simulink model "Telescope_model_PID"  (R2024b)
settings: Solver=ode4  StartTime=0.0  StopTime=SimulationTime  FixedStep=Tc  RelTol=1e-5
undefined symbols (not defined in the file): Arcs2Deg, Deg2Arcs, Kd_az, Kd_el, Ki_az, Ki_el, Kp_az, Kp_el, Kv, Prepocessor, Scenario, sgn, sysAz, sysEL, VonKarman
libraries: simulink x16
(part 2 of 2)

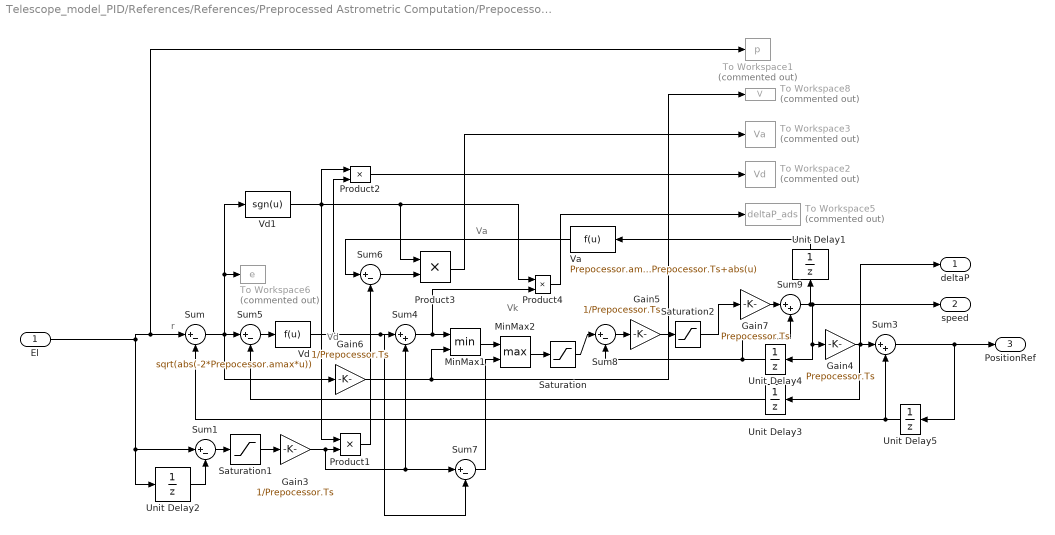
== system Telescope_model_PID/References/References/Preprocessed Astrometric Computation/Prepocessor Elavation/Prepocessor Elevation ==
  note: Vd
  note: Va
  note: Vk
  note: r
  El : Inport
  Gain3 : Gain  Gain=1/Prepocessor.Ts
  Gain4 : Gain  Gain=Prepocessor.Ts
  Gain5 : Gain  Gain=1/Prepocessor.Ts
  Gain6 : Gain  Gain=1/Prepocessor.Ts
  Gain7 : Gain  Gain=Prepocessor.Ts
  MinMax1 : MinMax  Inputs=2
  MinMax2 : MinMax  Function=max  Inputs=2
  Product{1..4} (4 alike) : Product
  Saturation : Saturate  UpperLimit=Prepocessor.vmax  LowerLimit=-Prepocessor.vmax
  Saturation1 : Saturate  UpperLimit=Prepocessor.vmax*Prepocessor.Ts  LowerLimit=-Prepocessor.vmax*Prepocessor.Ts
  Saturation2 : Saturate  UpperLimit=Prepocessor.amax  LowerLimit=-Prepocessor.amax
  Sum{,1,5..8} (6 alike) : Sum  Inputs=|+-
  Sum3 : Sum  Inputs=|++
  Sum4 : Sum  Inputs=|++
  Sum9 : Sum  Inputs=|++
  To Workspace1 : ToWorkspace  Commented=on  VariableName=p  SampleTime=-1
  To Workspace2 : ToWorkspace  Commented=on  VariableName=Vd  SampleTime=-1
  To Workspace3 : ToWorkspace  Commented=on  VariableName=Va  SampleTime=-1
  To Workspace5 : ToWorkspace  Commented=on  VariableName=deltaP_ads  SampleTime=-1
  To Workspace6 : ToWorkspace  Commented=on  VariableName=e  SampleTime=-1
  To Workspace8 : ToWorkspace  Commented=on  VariableName=V  SampleTime=-1
  Unit Delay{1..4} (4 alike) : UnitDelay  SampleTime=-1  HasFrameUpgradeWarning=on
  Unit Delay5 : UnitDelay  InitialCondition=Prepocessor.p0el  SampleTime=-1  HasFrameUpgradeWarning=on
  Va : Fcn  Expr=Prepocessor.amax*Prepocessor.Ts+abs(u)
  Vd : Fcn  Expr=sqrt(abs(-2*Prepocessor.amax*u))
  Vd1 : Fcn  Expr=sgn(u)
  deltaP : Outport
  speed : Outport  Port=2
  PositionRef : Outport  Port=3
  wires:
  Unit Delay5/1 -> Sum/2, Sum3/2
  Product4/1 -> To Workspace5/1
  El/1 -> Unit Delay2/1, Sum1/1, Sum/1, To Workspace1/1
  Product2/1 -> To Workspace2/1
  Product3/1 -> To Workspace3/1
  Vd/1 -> Product2/2, Sum7/2, Sum4/1
  Sum4/1 -> Product4/2, MinMax1/1
  Unit Delay3/1 -> Sum5/2
  Product1/1 -> Sum6/2
  Gain4/1 -> deltaP/1, Sum3/1, Unit Delay3/1
  Vd1/1 -> Product2/1, Product1/1, Product4/1, Product3/1
  Saturation2/1 -> Gain7/1
  Sum7/1 -> MinMax2/2
  Va/1 -> Sum6/1
  Sum1/1 -> Saturation1/1
  Sum/1 -> Sum5/1, Gain6/1, Vd1/1, To Workspace6/1
  Unit Delay2/1 -> Sum1/2
  Gain7/1 -> Sum9/1
  Sum9/1 -> speed/1, Unit Delay4/1, Gain4/1, Unit Delay1/1
  Unit Delay4/1 -> Sum8/2, Sum9/2
  Gain6/1 -> MinMax1/2, To Workspace8/1
  MinMax1/1 -> MinMax2/1
  Gain3/1 -> Sum7/1, Sum4/2, Product1/2
  Sum6/1 -> Product3/2
  Saturation1/1 -> Gain3/1
  Saturation/1 -> Sum8/1
  Sum8/1 -> Gain5/1
  Sum5/1 -> Vd/1
  MinMax2/1 -> Saturation/1
  Unit Delay1/1 -> Va/1
  Gain5/1 -> Saturation2/1
  Sum3/1 -> Unit Delay5/1, PositionRef/1

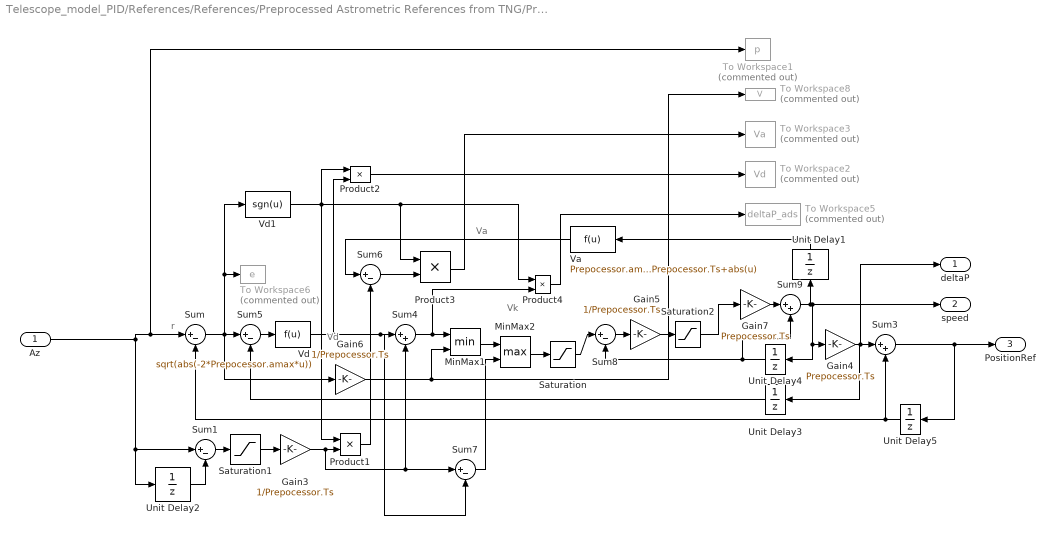
== system Telescope_model_PID/References/References/Preprocessed Astrometric References from TNG/Prepocessor Azimuth/Prepocessor Elevation ==
  note: Vd
  note: Va
  note: Vk
  note: r
  Az : Inport
  Gain3 : Gain  Gain=1/Prepocessor.Ts
  Gain4 : Gain  Gain=Prepocessor.Ts
  Gain5 : Gain  Gain=1/Prepocessor.Ts
  Gain6 : Gain  Gain=1/Prepocessor.Ts
  Gain7 : Gain  Gain=Prepocessor.Ts
  MinMax1 : MinMax  Inputs=2
  MinMax2 : MinMax  Function=max  Inputs=2
  Product{1..4} (4 alike) : Product
  Saturation : Saturate  UpperLimit=Prepocessor.vmax  LowerLimit=-Prepocessor.vmax
  Saturation1 : Saturate  UpperLimit=Prepocessor.vmax*Prepocessor.Ts  LowerLimit=-Prepocessor.vmax*Prepocessor.Ts
  Saturation2 : Saturate  UpperLimit=Prepocessor.amax  LowerLimit=-Prepocessor.amax
  Sum{,1,5..8} (6 alike) : Sum  Inputs=|+-
  Sum3 : Sum  Inputs=|++
  Sum4 : Sum  Inputs=|++
  Sum9 : Sum  Inputs=|++
  To Workspace1 : ToWorkspace  Commented=on  VariableName=p  SampleTime=-1
  To Workspace2 : ToWorkspace  Commented=on  VariableName=Vd  SampleTime=-1
  To Workspace3 : ToWorkspace  Commented=on  VariableName=Va  SampleTime=-1
  To Workspace5 : ToWorkspace  Commented=on  VariableName=deltaP_ads  SampleTime=-1
  To Workspace6 : ToWorkspace  Commented=on  VariableName=e  SampleTime=-1
  To Workspace8 : ToWorkspace  Commented=on  VariableName=V  SampleTime=-1
  Unit Delay{1..4} (4 alike) : UnitDelay  SampleTime=-1  HasFrameUpgradeWarning=on
  Unit Delay5 : UnitDelay  InitialCondition=Prepocessor.p0az  SampleTime=-1  HasFrameUpgradeWarning=on
  Va : Fcn  Expr=Prepocessor.amax*Prepocessor.Ts+abs(u)
  Vd : Fcn  Expr=sqrt(abs(-2*Prepocessor.amax*u))
  Vd1 : Fcn  Expr=sgn(u)
  deltaP : Outport
  speed : Outport  Port=2
  PositionRef : Outport  Port=3
  wires:
  Unit Delay5/1 -> Sum/2, Sum3/2
  Product4/1 -> To Workspace5/1
  Az/1 -> Unit Delay2/1, Sum1/1, Sum/1, To Workspace1/1
  Product2/1 -> To Workspace2/1
  Product3/1 -> To Workspace3/1
  Vd/1 -> Product2/2, Sum7/2, Sum4/1
  Sum4/1 -> Product4/2, MinMax1/1
  Unit Delay3/1 -> Sum5/2
  Product1/1 -> Sum6/2
  Gain4/1 -> deltaP/1, Sum3/1, Unit Delay3/1
  Vd1/1 -> Product2/1, Product1/1, Product4/1, Product3/1
  Saturation2/1 -> Gain7/1
  Sum7/1 -> MinMax2/2
  Va/1 -> Sum6/1
  Sum1/1 -> Saturation1/1
  Sum/1 -> Sum5/1, Gain6/1, Vd1/1, To Workspace6/1
  Unit Delay2/1 -> Sum1/2
  Gain7/1 -> Sum9/1
  Sum9/1 -> speed/1, Unit Delay4/1, Gain4/1, Unit Delay1/1
  Unit Delay4/1 -> Sum8/2, Sum9/2
  Gain6/1 -> MinMax1/2, To Workspace8/1
  MinMax1/1 -> MinMax2/1
  Gain3/1 -> Sum7/1, Sum4/2, Product1/2
  Sum6/1 -> Product3/2
  Saturation1/1 -> Gain3/1
  Saturation/1 -> Sum8/1
  Sum8/1 -> Gain5/1
  Sum5/1 -> Vd/1
  MinMax2/1 -> Saturation/1
  Unit Delay1/1 -> Va/1
  Gain5/1 -> Saturation2/1
  Sum3/1 -> Unit Delay5/1, PositionRef/1

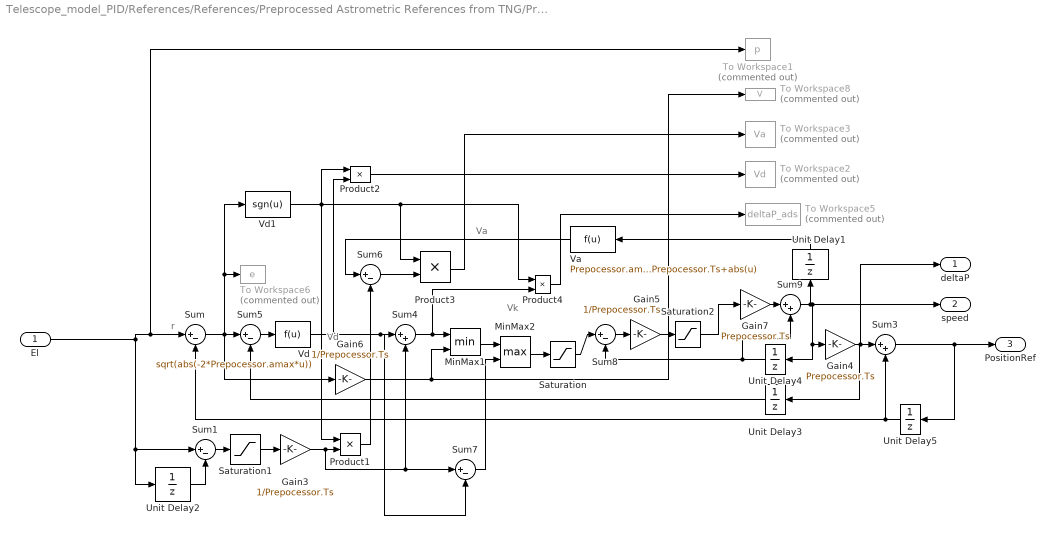
== system Telescope_model_PID/References/References/Preprocessed Astrometric References from TNG/Prepocessor Elavation/Prepocessor Elevation ==
  note: Vd
  note: Va
  note: Vk
  note: r
  El : Inport
  Gain3 : Gain  Gain=1/Prepocessor.Ts
  Gain4 : Gain  Gain=Prepocessor.Ts
  Gain5 : Gain  Gain=1/Prepocessor.Ts
  Gain6 : Gain  Gain=1/Prepocessor.Ts
  Gain7 : Gain  Gain=Prepocessor.Ts
  MinMax1 : MinMax  Inputs=2
  MinMax2 : MinMax  Function=max  Inputs=2
  Product{1..4} (4 alike) : Product
  Saturation : Saturate  UpperLimit=Prepocessor.vmax  LowerLimit=-Prepocessor.vmax
  Saturation1 : Saturate  UpperLimit=Prepocessor.vmax*Prepocessor.Ts  LowerLimit=-Prepocessor.vmax*Prepocessor.Ts
  Saturation2 : Saturate  UpperLimit=Prepocessor.amax  LowerLimit=-Prepocessor.amax
  Sum{,1,5..8} (6 alike) : Sum  Inputs=|+-
  Sum3 : Sum  Inputs=|++
  Sum4 : Sum  Inputs=|++
  Sum9 : Sum  Inputs=|++
  To Workspace1 : ToWorkspace  Commented=on  VariableName=p  SampleTime=-1
  To Workspace2 : ToWorkspace  Commented=on  VariableName=Vd  SampleTime=-1
  To Workspace3 : ToWorkspace  Commented=on  VariableName=Va  SampleTime=-1
  To Workspace5 : ToWorkspace  Commented=on  VariableName=deltaP_ads  SampleTime=-1
  To Workspace6 : ToWorkspace  Commented=on  VariableName=e  SampleTime=-1
  To Workspace8 : ToWorkspace  Commented=on  VariableName=V  SampleTime=-1
  Unit Delay{1..4} (4 alike) : UnitDelay  SampleTime=-1  HasFrameUpgradeWarning=on
  Unit Delay5 : UnitDelay  InitialCondition=Prepocessor.p0el  SampleTime=-1  HasFrameUpgradeWarning=on
  Va : Fcn  Expr=Prepocessor.amax*Prepocessor.Ts+abs(u)
  Vd : Fcn  Expr=sqrt(abs(-2*Prepocessor.amax*u))
  Vd1 : Fcn  Expr=sgn(u)
  deltaP : Outport
  speed : Outport  Port=2
  PositionRef : Outport  Port=3
  wires:
  Unit Delay5/1 -> Sum/2, Sum3/2
  Product4/1 -> To Workspace5/1
  El/1 -> Unit Delay2/1, Sum1/1, Sum/1, To Workspace1/1
  Product2/1 -> To Workspace2/1
  Product3/1 -> To Workspace3/1
  Vd/1 -> Product2/2, Sum7/2, Sum4/1
  Sum4/1 -> Product4/2, MinMax1/1
  Unit Delay3/1 -> Sum5/2
  Product1/1 -> Sum6/2
  Gain4/1 -> deltaP/1, Sum3/1, Unit Delay3/1
  Vd1/1 -> Product2/1, Product1/1, Product4/1, Product3/1
  Saturation2/1 -> Gain7/1
  Sum7/1 -> MinMax2/2
  Va/1 -> Sum6/1
  Sum1/1 -> Saturation1/1
  Sum/1 -> Sum5/1, Gain6/1, Vd1/1, To Workspace6/1
  Unit Delay2/1 -> Sum1/2
  Gain7/1 -> Sum9/1
  Sum9/1 -> speed/1, Unit Delay4/1, Gain4/1, Unit Delay1/1
  Unit Delay4/1 -> Sum8/2, Sum9/2
  Gain6/1 -> MinMax1/2, To Workspace8/1
  MinMax1/1 -> MinMax2/1
  Gain3/1 -> Sum7/1, Sum4/2, Product1/2
  Sum6/1 -> Product3/2
  Saturation1/1 -> Gain3/1
  Saturation/1 -> Sum8/1
  Sum8/1 -> Gain5/1
  Sum5/1 -> Vd/1
  MinMax2/1 -> Saturation/1
  Unit Delay1/1 -> Va/1
  Gain5/1 -> Saturation2/1
  Sum3/1 -> Unit Delay5/1, PositionRef/1

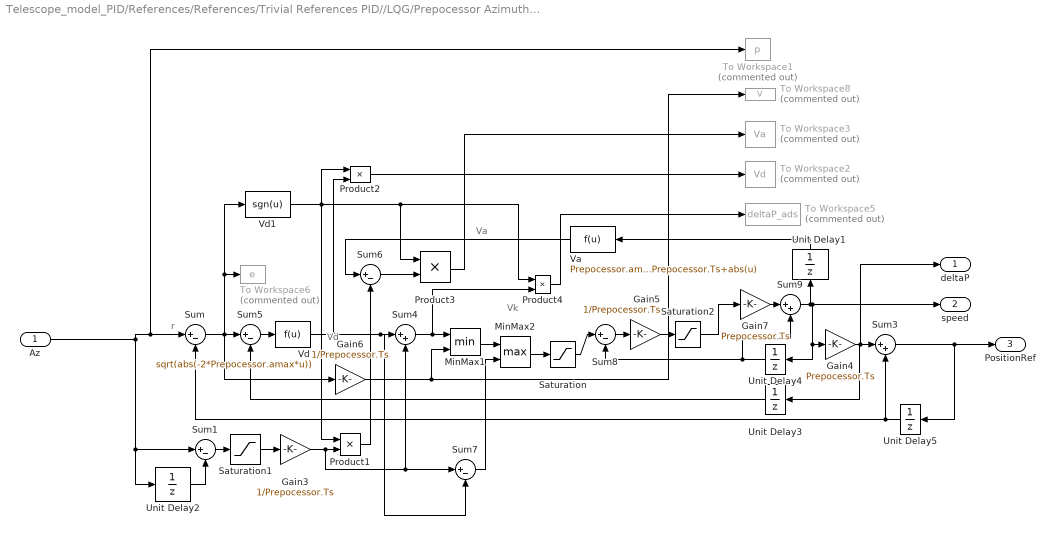
== system Telescope_model_PID/References/References/Trivial References PID//LQG/Prepocessor Azimuth/Prepocessor Elevation ==
  note: Vd
  note: Va
  note: Vk
  note: r
  Az : Inport
  Gain3 : Gain  Gain=1/Prepocessor.Ts
  Gain4 : Gain  Gain=Prepocessor.Ts
  Gain5 : Gain  Gain=1/Prepocessor.Ts
  Gain6 : Gain  Gain=1/Prepocessor.Ts
  Gain7 : Gain  Gain=Prepocessor.Ts
  MinMax1 : MinMax  Inputs=2
  MinMax2 : MinMax  Function=max  Inputs=2
  Product{1..4} (4 alike) : Product
  Saturation : Saturate  UpperLimit=Prepocessor.vmax  LowerLimit=-Prepocessor.vmax
  Saturation1 : Saturate  UpperLimit=Prepocessor.vmax*Prepocessor.Ts  LowerLimit=-Prepocessor.vmax*Prepocessor.Ts
  Saturation2 : Saturate  UpperLimit=Prepocessor.amax  LowerLimit=-Prepocessor.amax
  Sum{,1,5..8} (6 alike) : Sum  Inputs=|+-
  Sum3 : Sum  Inputs=|++
  Sum4 : Sum  Inputs=|++
  Sum9 : Sum  Inputs=|++
  To Workspace1 : ToWorkspace  Commented=on  VariableName=p  SampleTime=-1
  To Workspace2 : ToWorkspace  Commented=on  VariableName=Vd  SampleTime=-1
  To Workspace3 : ToWorkspace  Commented=on  VariableName=Va  SampleTime=-1
  To Workspace5 : ToWorkspace  Commented=on  VariableName=deltaP_ads  SampleTime=-1
  To Workspace6 : ToWorkspace  Commented=on  VariableName=e  SampleTime=-1
  To Workspace8 : ToWorkspace  Commented=on  VariableName=V  SampleTime=-1
  Unit Delay{1..4} (4 alike) : UnitDelay  SampleTime=-1  HasFrameUpgradeWarning=on
  Unit Delay5 : UnitDelay  InitialCondition=Prepocessor.p0az  SampleTime=-1  HasFrameUpgradeWarning=on
  Va : Fcn  Expr=Prepocessor.amax*Prepocessor.Ts+abs(u)
  Vd : Fcn  Expr=sqrt(abs(-2*Prepocessor.amax*u))
  Vd1 : Fcn  Expr=sgn(u)
  deltaP : Outport
  speed : Outport  Port=2
  PositionRef : Outport  Port=3
  wires:
  Unit Delay5/1 -> Sum/2, Sum3/2
  Product4/1 -> To Workspace5/1
  Az/1 -> Unit Delay2/1, Sum1/1, Sum/1, To Workspace1/1
  Product2/1 -> To Workspace2/1
  Product3/1 -> To Workspace3/1
  Vd/1 -> Product2/2, Sum7/2, Sum4/1
  Sum4/1 -> Product4/2, MinMax1/1
  Unit Delay3/1 -> Sum5/2
  Product1/1 -> Sum6/2
  Gain4/1 -> deltaP/1, Sum3/1, Unit Delay3/1
  Vd1/1 -> Product2/1, Product1/1, Product4/1, Product3/1
  Saturation2/1 -> Gain7/1
  Sum7/1 -> MinMax2/2
  Va/1 -> Sum6/1
  Sum1/1 -> Saturation1/1
  Sum/1 -> Sum5/1, Gain6/1, Vd1/1, To Workspace6/1
  Unit Delay2/1 -> Sum1/2
  Gain7/1 -> Sum9/1
  Sum9/1 -> speed/1, Unit Delay4/1, Gain4/1, Unit Delay1/1
  Unit Delay4/1 -> Sum8/2, Sum9/2
  Gain6/1 -> MinMax1/2, To Workspace8/1
  MinMax1/1 -> MinMax2/1
  Gain3/1 -> Sum7/1, Sum4/2, Product1/2
  Sum6/1 -> Product3/2
  Saturation1/1 -> Gain3/1
  Saturation/1 -> Sum8/1
  Sum8/1 -> Gain5/1
  Sum5/1 -> Vd/1
  MinMax2/1 -> Saturation/1
  Unit Delay1/1 -> Va/1
  Gain5/1 -> Saturation2/1
  Sum3/1 -> Unit Delay5/1, PositionRef/1

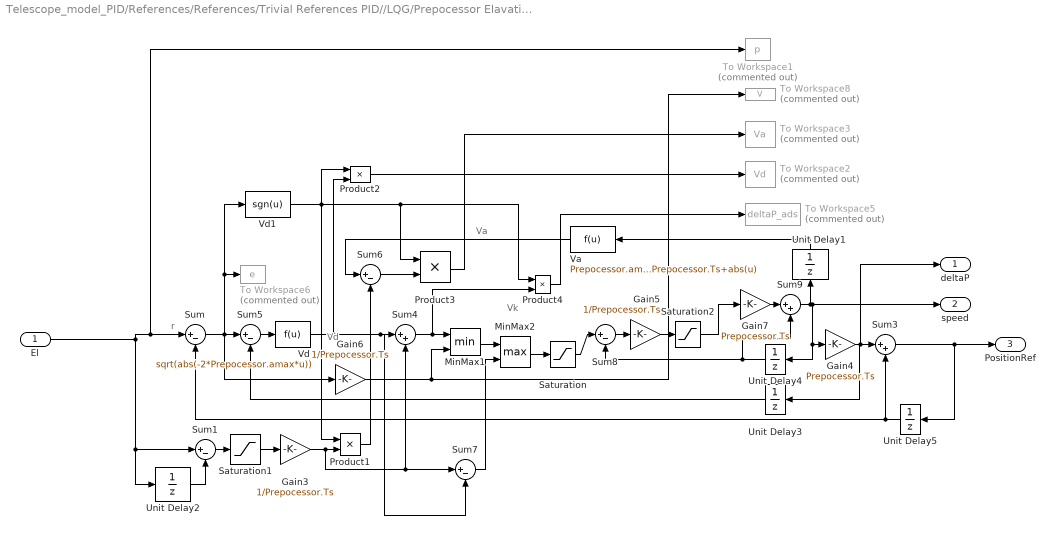
== system Telescope_model_PID/References/References/Trivial References PID//LQG/Prepocessor Elavation/Prepocessor Elevation ==
  note: Vd
  note: Va
  note: Vk
  note: r
  El : Inport
  Gain3 : Gain  Gain=1/Prepocessor.Ts
  Gain4 : Gain  Gain=Prepocessor.Ts
  Gain5 : Gain  Gain=1/Prepocessor.Ts
  Gain6 : Gain  Gain=1/Prepocessor.Ts
  Gain7 : Gain  Gain=Prepocessor.Ts
  MinMax1 : MinMax  Inputs=2
  MinMax2 : MinMax  Function=max  Inputs=2
  Product{1..4} (4 alike) : Product
  Saturation : Saturate  UpperLimit=Prepocessor.vmax  LowerLimit=-Prepocessor.vmax
  Saturation1 : Saturate  UpperLimit=Prepocessor.vmax*Prepocessor.Ts  LowerLimit=-Prepocessor.vmax*Prepocessor.Ts
  Saturation2 : Saturate  UpperLimit=Prepocessor.amax  LowerLimit=-Prepocessor.amax
  Sum{,1,5..8} (6 alike) : Sum  Inputs=|+-
  Sum3 : Sum  Inputs=|++
  Sum4 : Sum  Inputs=|++
  Sum9 : Sum  Inputs=|++
  To Workspace1 : ToWorkspace  Commented=on  VariableName=p  SampleTime=-1
  To Workspace2 : ToWorkspace  Commented=on  VariableName=Vd  SampleTime=-1
  To Workspace3 : ToWorkspace  Commented=on  VariableName=Va  SampleTime=-1
  To Workspace5 : ToWorkspace  Commented=on  VariableName=deltaP_ads  SampleTime=-1
  To Workspace6 : ToWorkspace  Commented=on  VariableName=e  SampleTime=-1
  To Workspace8 : ToWorkspace  Commented=on  VariableName=V  SampleTime=-1
  Unit Delay{1..4} (4 alike) : UnitDelay  SampleTime=-1  HasFrameUpgradeWarning=on
  Unit Delay5 : UnitDelay  InitialCondition=Prepocessor.p0el  SampleTime=-1  HasFrameUpgradeWarning=on
  Va : Fcn  Expr=Prepocessor.amax*Prepocessor.Ts+abs(u)
  Vd : Fcn  Expr=sqrt(abs(-2*Prepocessor.amax*u))
  Vd1 : Fcn  Expr=sgn(u)
  deltaP : Outport
  speed : Outport  Port=2
  PositionRef : Outport  Port=3
  wires:
  Unit Delay5/1 -> Sum/2, Sum3/2
  Product4/1 -> To Workspace5/1
  El/1 -> Unit Delay2/1, Sum1/1, Sum/1, To Workspace1/1
  Product2/1 -> To Workspace2/1
  Product3/1 -> To Workspace3/1
  Vd/1 -> Product2/2, Sum7/2, Sum4/1
  Sum4/1 -> Product4/2, MinMax1/1
  Unit Delay3/1 -> Sum5/2
  Product1/1 -> Sum6/2
  Gain4/1 -> deltaP/1, Sum3/1, Unit Delay3/1
  Vd1/1 -> Product2/1, Product1/1, Product4/1, Product3/1
  Saturation2/1 -> Gain7/1
  Sum7/1 -> MinMax2/2
  Va/1 -> Sum6/1
  Sum1/1 -> Saturation1/1
  Sum/1 -> Sum5/1, Gain6/1, Vd1/1, To Workspace6/1
  Unit Delay2/1 -> Sum1/2
  Gain7/1 -> Sum9/1
  Sum9/1 -> speed/1, Unit Delay4/1, Gain4/1, Unit Delay1/1
  Unit Delay4/1 -> Sum8/2, Sum9/2
  Gain6/1 -> MinMax1/2, To Workspace8/1
  MinMax1/1 -> MinMax2/1
  Gain3/1 -> Sum7/1, Sum4/2, Product1/2
  Sum6/1 -> Product3/2
  Saturation1/1 -> Gain3/1
  Saturation/1 -> Sum8/1
  Sum8/1 -> Gain5/1
  Sum5/1 -> Vd/1
  MinMax2/1 -> Saturation/1
  Unit Delay1/1 -> Va/1
  Gain5/1 -> Saturation2/1
  Sum3/1 -> Unit Delay5/1, PositionRef/1

== system Telescope_model_PID/Telescope Model/Azimuth Model 50 deg/Noise Model/Von Karman Torque PSD/Sv ==
  note: Output PSD
  note: Denominator
  f : Inport
  Add : Sum
  Constant : Constant
  Constant1 : Constant  Value=5/6
  Constant2 : Constant  Value=4*(VonKarman.I*VonKarman.v_mean)^2*(VonKarman.L/VonKarman.v_mean)
  Divide : Product  Inputs=*/
  Gain : Gain  Gain=(1.339*VonKarman.L)/VonKarman.v_mean
  Square : Math  Operator=square
  Square1 : Math  Operator=pow
  Out_Sv : Outport
  wires:
  Constant/1 -> Add/1
  f/1 -> Gain/1
  Gain/1 -> Square/1
  Square/1 -> Add/2
  Add/1 -> Square1/1
  Constant1/1 -> Square1/2
  [DEN] -> Divide/2
  Square1/1 -> [DEN]
  Constant2/1 -> Divide/1
  Divide/1 -> Out_Sv/1

== system Telescope_model_PID/Telescope Model/Azimuth Model 50 deg/Noise Model/Von Karman Torque PSD/X ==
  note: X PSD
  f : Inport
  Add : Sum
  Constant : Constant
  Constant1 : Constant  Value=4/3
  Constant2 : Constant
  Divide : Product  Inputs=*/
  Gain : Gain  Gain=2*sqrt(VonKarman.A)/VonKarman.v_mean
  Square1 : Math  Operator=pow
  Out_X : Outport
  wires:
  Constant/1 -> Add/1
  f/1 -> Gain/1
  Constant1/1 -> Square1/2
  Constant2/1 -> Divide/1
  Divide/1 -> Out_X/1
  Add/1 -> Divide/2
  Gain/1 -> Square1/1
  Square1/1 -> Add/2

== system Telescope_model_PID/Telescope Model/Elevation Model/Noise Model/Von Karman Torque PSD/Sv ==
  note: Output PSD
  note: Denominator
  f : Inport
  Add : Sum
  Constant : Constant
  Constant1 : Constant  Value=5/6
  Constant2 : Constant  Value=4*(VonKarman.I*VonKarman.v_mean)^2*(VonKarman.L/VonKarman.v_mean)
  Divide : Product  Inputs=*/
  Gain : Gain  Gain=(1.339*VonKarman.L)/VonKarman.v_mean
  Square : Math  Operator=square
  Square1 : Math  Operator=pow
  Out_Sv : Outport
  wires:
  Constant/1 -> Add/1
  f/1 -> Gain/1
  Gain/1 -> Square/1
  Square/1 -> Add/2
  Add/1 -> Square1/1
  Constant1/1 -> Square1/2
  [DEN] -> Divide/2
  Square1/1 -> [DEN]
  Constant2/1 -> Divide/1
  Divide/1 -> Out_Sv/1

== system Telescope_model_PID/Telescope Model/Elevation Model/Noise Model/Von Karman Torque PSD/X ==
  note: X PSD
  f : Inport
  Add : Sum
  Constant : Constant
  Constant1 : Constant  Value=4/3
  Constant2 : Constant
  Divide : Product  Inputs=*/
  Gain : Gain  Gain=2*sqrt(VonKarman.A)/VonKarman.v_mean
  Square1 : Math  Operator=pow
  Out_X : Outport
  wires:
  Constant/1 -> Add/1
  f/1 -> Gain/1
  Constant1/1 -> Square1/2
  Constant2/1 -> Divide/1
  Divide/1 -> Out_X/1
  Add/1 -> Divide/2
  Gain/1 -> Square1/1
  Square1/1 -> Add/2

== matlab function Telescope_model_PID/References/References/Astrometric Computation/MATLAB Function ==
  data: clo input; Time input; RAhh input; RAmm input; RAss input; DECdd input; DECmm input; DECss input; Latitude input; Longitude input; VLT input; Az output; Alt output
function [Az, Alt] = astroCalc(clo, Time, RAhh, RAmm, RAss, DECdd, DECmm, DECss, Latitude, Longitude, VLT)

  
   %% Legge l'orario del clock di sistema
   Y = Time(1);
   M = Time(2);
   D = Time(3);
   H = Time(4);
   MN = Time(5);
   S = Time(6);
   S = S + clo;
   if S > 60
       S = 0;
       MN = MN+1;
   end
   if MN>60
       MN = 00;
       H = H+1;
   end
   if H>24
       H = 1;
       D = D+1;
   end
   if D>31
       D = 0;
       M = M+1;
   end
   if M>12
       M = 1;
       Y = Y+1;
   end

   % Calcola data e ora
   year   = Y;
   month  = M;
   day    = D;
   PCHour = H;
   hour   = PCHour-1; % UT
   % Correzione brutale per ora legale. Funziona... quasi sempre.
   if month >=4 & month<=10
       hour = hour - 1;
   end
   min = MN;
   sec = S;
   
   %% Aggiunge al tempo di sistema il clock della simulazione Simulink
   sec     = sec + clo;     % aggiungo i secondi del tempo di simulazione
   minplus = floor(sec/60); % calcolo il numero di minuti da aggiungere
   sec     = mod(sec,60);   % limito i secondi nel range giusto
   min     = min + minplus; % aggiungo i minuti
   hplus   = floor(min/60); % calcolo il numero di ore da aggiungere
   min     = mod(min,60);   % limito i minuti nel range giusto
   hour    = hour + hplus;  % aggiungo le ore  
   hour    = mod(hour,24);  % limito le ore nel range giusto
    
   %% Calcola RA,DEC
   RA=(RAhh+RAmm/60+RAss/3600)*360/24;
   Dec=DECdd+DECmm/60+DECss/3600;

   %% Calcoli astrometrici
   JD = floor(365.25*(year + 4716.0)) + floor(30.6001*( month + 1.0)) + 2.0 - ...
    floor(year/100.0) + floor(floor(year/100.0 )/4.0) + day - 1524.5 + ...
    (hour + min/60 + sec/3600)/24;
   D = JD - 2451543.5;
   w = 282.9404 + 4.70935e-5*D;
   M = mod(356.0470 + 0.9856002585*D,360);
   L = w + M;
   GMST0 = mod(L + 180,360)/15;
   UT_hour = hour + min/60 + sec/3600;
   SiderealTime = GMST0 + UT_hour + Longitude/15;
      
   lst = SiderealTime;
   if lst > 24
    lst=lst-24;
   end

   lsth=floor(lst);
   lstm=floor((lst-floor(lst))*60);
   lsts=((lst-floor(lst))*60-floor((lst-floor(lst))*60))*60;

   HourAngle = (SiderealTime*360/24 - RA);

% Calcolo alternativo equivalente   
% A = cosd(HourAngle)*cosd(Dec)*cosd(90 - Latitude) - sind(Dec)*sind(90 - Latitude);
% B = sind(HourAngle)*cosd(Dec);
% C = cosd(HourAngle)*cosd(Dec)*sind(90 - Latitude) + sind(Dec)*cosd(90 - Latitude);
% Az1 = atan2(B,A)*180/pi + 180;
% Alt1 = asin(C)*180/pi;
% if VLT==1
%     Az1 = -(Az1+180);
% end
 
      
   hRad   = HourAngle*pi/180;
   DECRad = Dec*pi/180;
   phiRad = Latitude*pi/180;

%https://en.wikipedia.org/wiki/Celestial_coordinate_system
   x = -sin(phiRad)*cos(DECRad).*cos(hRad)+cos(phiRad)*sin(DECRad);
   y = cos(DECRad).*sin(hRad);
   Az  = mod(-atan2(y,x)*180/pi,360);
   
% convenzione VLT! South=0; verso positivo: counterclockwise
% normalmente invece North=0; verso positivo: clockwise
   if VLT==1
    Az = -(Az+180);
   end
   
   Alt = asin(sin(phiRad)*sin(DECRad)+cos(phiRad)*cos(DECRad).*cos(hRad))*180/pi;

% https://en.wikipedia.org/wiki/Parallactic_angle
   yr = sin(hRad);
   xr = cos(DECRad)*tan(phiRad)-sin(DECRad).*cos(hRad);
   Rot = atan2(yr,xr)*180/pi;

== matlab function Telescope_model_PID/References/References/Preprocessed Astrometric Computation/MATLAB Function ==
  data: clo input; Time input; RAhh input; RAmm input; RAss input; DECdd input; DECmm input; DECss input; Latitude input; Longitude input; VLT input; Az output; Alt output
function [Az, Alt] = astroCalc(clo, Time, RAhh, RAmm, RAss, DECdd, DECmm, DECss, Latitude, Longitude, VLT)

  
   %% Legge l'orario del clock di sistema
   Y = Time(1);
   M = Time(2);
   D = Time(3);
   H = Time(4);
   MN = Time(5);
   S = Time(6);
   S = S + clo;
   if S > 60
       S = 0;
       MN = MN+1;
   end
   if MN>60
       MN = 00;
       H = H+1;
   end
   if H>24
       H = 1;
       D = D+1;
   end
   if D>31
       D = 0;
       M = M+1;
   end
   if M>12
       M = 1;
       Y = Y+1;
   end

   % Calcola data e ora
   year   = Y;
   month  = M;
   day    = D;
   PCHour = H;
   hour   = PCHour-1; % UT
   % Correzione brutale per ora legale. Funziona... quasi sempre.
   if month >=4 & month<=10
       hour = hour - 1;
   end
   min = MN;
   sec = S;
   
   %% Aggiunge al tempo di sistema il clock della simulazione Simulink
   sec     = sec + clo;     % aggiungo i secondi del tempo di simulazione
   minplus = floor(sec/60); % calcolo il numero di minuti da aggiungere
   sec     = mod(sec,60);   % limito i secondi nel range giusto
   min     = min + minplus; % aggiungo i minuti
   hplus   = floor(min/60); % calcolo il numero di ore da aggiungere
   min     = mod(min,60);   % limito i minuti nel range giusto
   hour    = hour + hplus;  % aggiungo le ore  
   hour    = mod(hour,24);  % limito le ore nel range giusto
    
   %% Calcola RA,DEC
   RA=(RAhh+RAmm/60+RAss/3600)*360/24;
   Dec=DECdd+DECmm/60+DECss/3600;

   %% Calcoli astrometrici
   JD = floor(365.25*(year + 4716.0)) + floor(30.6001*( month + 1.0)) + 2.0 - ...
    floor(year/100.0) + floor(floor(year/100.0 )/4.0) + day - 1524.5 + ...
    (hour + min/60 + sec/3600)/24;
   D = JD - 2451543.5;
   w = 282.9404 + 4.70935e-5*D;
   M = mod(356.0470 + 0.9856002585*D,360);
   L = w + M;
   GMST0 = mod(L + 180,360)/15;
   UT_hour = hour + min/60 + sec/3600;
   SiderealTime = GMST0 + UT_hour + Longitude/15;
      
   lst = SiderealTime;
   if lst > 24
    lst=lst-24;
   end

   lsth=floor(lst);
   lstm=floor((lst-floor(lst))*60);
   lsts=((lst-floor(lst))*60-floor((lst-floor(lst))*60))*60;

   HourAngle = (SiderealTime*360/24 - RA);

% Calcolo alternativo equivalente   
% A = cosd(HourAngle)*cosd(Dec)*cosd(90 - Latitude) - sind(Dec)*sind(90 - Latitude);
% B = sind(HourAngle)*cosd(Dec);
% C = cosd(HourAngle)*cosd(Dec)*sind(90 - Latitude) + sind(Dec)*cosd(90 - Latitude);
% Az1 = atan2(B,A)*180/pi + 180;
% Alt1 = asin(C)*180/pi;
% if VLT==1
%     Az1 = -(Az1+180);
% end
 
      
   hRad   = HourAngle*pi/180;
   DECRad = Dec*pi/180;
   phiRad = Latitude*pi/180;

%https://en.wikipedia.org/wiki/Celestial_coordinate_system
   x = -sin(phiRad)*cos(DECRad).*cos(hRad)+cos(phiRad)*sin(DECRad);
   y = cos(DECRad).*sin(hRad);
   Az  = mod(-atan2(y,x)*180/pi,360);
   
% convenzione VLT! South=0; verso positivo: counterclockwise
% normalmente invece North=0; verso positivo: clockwise
   if VLT==1
    Az = -(Az+180);
   end
   
   Alt = asin(sin(phiRad)*sin(DECRad)+cos(phiRad)*cos(DECRad).*cos(hRad))*180/pi;

% https://en.wikipedia.org/wiki/Parallactic_angle
   yr = sin(hRad);
   xr = cos(DECRad)*tan(phiRad)-sin(DECRad).*cos(hRad);
   Rot = atan2(yr,xr)*180/pi;
